simulink model "parameter_and_set_adaptation"  (R2020a)
settings: Solver=FixedStepAuto  StartTime=0.0  StopTime=ts  FixedStep=0.001  RelTol=1e-3
values from neighbouring files (symbols this model uses):
  eta = zeros(6,nt+1)    [run_Adaptive_Robust_MPCA.m]
  omega = zeros(size(x,1),size(theta,1),nt+1)    [run_Adaptive_Robust_MPCA.m]
  Q = zeros(size(Q0,1),size(Q0,2),nt+1)    [run_Adaptive_Robust_MPCA.m]
  thetaHat = zeros(3,nt+1)    [run_Adaptive_Robust_MPCA.m]
  V_e_eta = zeros(nt+1,1)    [run_Adaptive_Robust_MPCA.m]
  x = zeros(6,nt+1)    [run_Adaptive_Robust_MPCA.m]
  xHat = zeros(6,nt+1)    [run_Adaptive_Robust_MPCA.m]
undefined symbols (not defined in the file or in its folder): gamma, i, Ixx, Iyy, Izz, K, theta, z_theta0
settings Model: Creator=12894  LastModifiedBy=Maxwell
settings DebuggingCC: ArithmeticOperatorsInVariantConditions=warning
settings SFSimCC: CustomCodeUndefinedFunction=UseInterfaceOnly
settings CodeAppCC: StateflowObjectComments=on

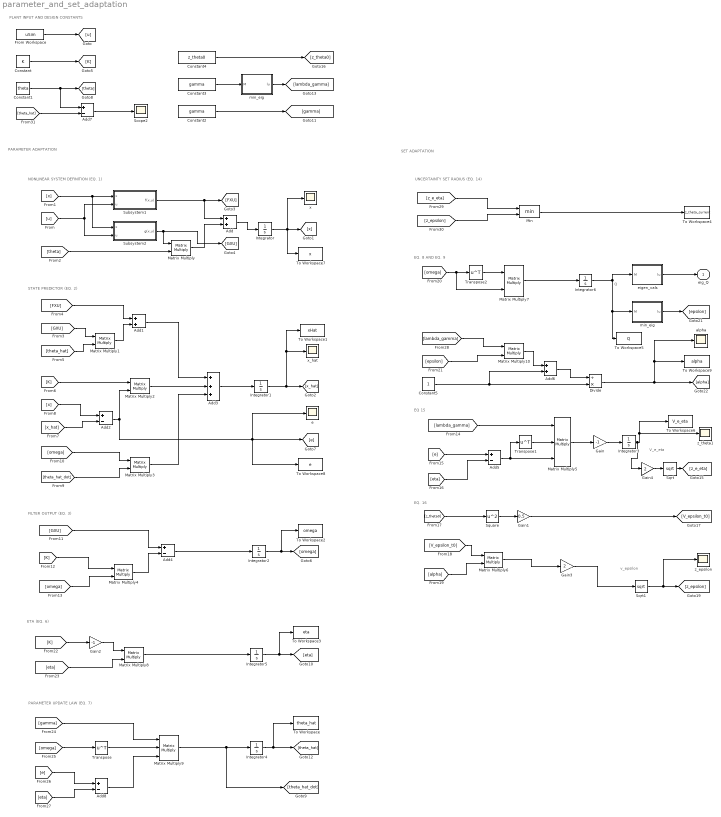
== system parameter_and_set_adaptation ==
  note: Q
  note: v_epsilon
  note: V_e_eta
  note: SET ADAPTATION
  note: UNCERTAINTY SET RADIUS (EQ. 14)
  note: EQ. 8 AND EQ. 9
  note: EQ. 16
  note: EQ 15
  note: PARAMETER ADAPTATION
  note: ETA (EQ. 6)
  note: PARAMETER UPDATE LAW (EQ. 7)
  note: FILTER OUTPUT (EQ. 3)
  note: STATE PREDICTOR (EQ. 2)
  note: NONLINEAR SYSTEM DEFINITION (EQ. 1)
  note: PLANT INPUT AND DESIGN CONSTANTS
  Add : Sum
  Add1 : Sum
  Add{2,4..5,7..8} (5 alike) : Sum  Inputs=+-
  Add3 : Sum  Inputs=+++
  Add6 : Sum
  Constant : Constant  Value=K
  Constant1 : Constant  Value=theta
  Constant2 : Constant  Value=gamma
  Constant3 : Constant  Value=gamma
  Constant4 : Constant  Value=z_theta0
  Constant5 : Constant
  Divide : Product  Inputs=/*
  From Workspace : FromWorkspace  VariableName=uSim
  Gain : Gain  Gain=-1
  Gain1 : Gain  Gain=0.5
  Gain2 : Gain  Gain=-1
  Gain3 : Gain  Gain=2
  Gain4 : Gain  Gain=2
  Integrator : Integrator  InitialCondition=x(:,i)
  Integrator1 : Integrator  InitialCondition=xHat(:,i)
  Integrator2 : Integrator  InitialCondition=omega(:,:,i)
  Integrator3 : Integrator  InitialCondition=V_e_eta(i)
  Integrator4 : Integrator  InitialCondition=thetaHat(:,i)
  Integrator5 : Integrator  InitialCondition=eta(:,i)
  Integrator6 : Integrator  InitialCondition=Q(:,:,i)
  Matrix Multiply{,1..4,6..8,10} (9 alike) : Product  Multiplication=Matrix(*)
  Matrix Multiply5 : Product  Inputs=3  Multiplication=Matrix(*)
  Matrix Multiply9 : Product  Inputs=3  Multiplication=Matrix(*)
  Min : MinMax  Inputs=2
  Scope2 : Scope
  Sqrt : Sqrt  SaturateOnIntegerOverflow=on
  Sqrt1 : Sqrt  SaturateOnIntegerOverflow=on
  Square : Math  Operator=square  SignedPower=on  SaturateOnIntegerOverflow=on
  Subsystem1 : Subsystem
  Subsystem2 : Subsystem
  To Workspace : ToWorkspace  VariableName=theta_hat  SaveFormat=Timeseries  SampleTime=-1
  To Workspace1 : ToWorkspace  VariableName=xHat  SaveFormat=Timeseries  SampleTime=-1
  To Workspace2 : ToWorkspace  VariableName=omega  SaveFormat=Timeseries  SampleTime=-1
  To Workspace3 : ToWorkspace  VariableName=eta  SaveFormat=Timeseries  SampleTime=-1
  To Workspace4 : ToWorkspace  VariableName=z_theta_current  SaveFormat=Timeseries  SampleTime=-1
  To Workspace5 : ToWorkspace  VariableName=Q  SaveFormat=Timeseries  SampleTime=-1
  To Workspace6 : ToWorkspace  VariableName=V_e_eta  SaveFormat=Timeseries  SampleTime=-1
  To Workspace7 : ToWorkspace  VariableName=x  SaveFormat=Timeseries  SampleTime=-1
  To Workspace8 : ToWorkspace  VariableName=e  SaveFormat=Timeseries  SampleTime=-1
  To Workspace9 : ToWorkspace  VariableName=alpha  SaveFormat=Timeseries  SampleTime=-1
  Transpose : Math  Operator=transpose  SignedPower=on  SaturateOnIntegerOverflow=on
  Transpose1 : Math  Operator=transpose  SignedPower=on  SaturateOnIntegerOverflow=on
  Transpose2 : Math  Operator=transpose  SignedPower=on  SaturateOnIntegerOverflow=on
  alpha : Scope
  e : Scope
  eigen_vals : MATLAB Function  TreatAsAtomicUnit=on
  min_eig : MATLAB Function  TreatAsAtomicUnit=on
  "min_eig " : MATLAB Function  TreatAsAtomicUnit=on
  x : Scope
  x_hat : Scope
  z_epsilon : Scope
  z_theta1 : Scope
  eig_Q : Outport  VectorParamsAs1DForOutWhenUnconnected=off
  wires:
  From Workspace/1 -> [u]
  [u] -> Subsystem1/2(u), Subsystem2/2(u)
  [x] -> Subsystem2/1(x), Subsystem1/1(x)
  Subsystem2/1(g(x,u)) -> [GXU], Matrix Multiply/1
  [theta] -> Matrix Multiply/2
  Subsystem1/1(f(x,u)) -> [FXU], Add/1
  Matrix Multiply/1 -> Add/2
  Integrator/1 -> To Workspace7/1, x/1, [x]
  Add/1 -> Integrator/1
  Matrix Multiply1/1 -> Add1/2
  [theta_hat] -> Matrix Multiply1/2
  Integrator1/1 -> To Workspace1/1, x_hat/1, [x_hat]
  [GXU] -> Matrix Multiply1/1
  [FXU] -> Add1/1
  [K] -> Matrix Multiply2/1
  Constant/1 -> [K]
  [x] -> Add2/1
  [x_hat] -> Add2/2
  Add2/1 -> To Workspace8/1, e/1, [e], Matrix Multiply2/2
  [omega] -> Matrix Multiply3/1
  [theta_hat_dot] -> Matrix Multiply3/2
  Add1/1 -> Add3/1
  Matrix Multiply2/1 -> Add3/2
  Matrix Multiply3/1 -> Add3/3
  Add3/1 -> Integrator1/1
  Integrator2/1 -> To Workspace2/1, [omega]
  [K] -> Matrix Multiply4/1
  [omega] -> Matrix Multiply4/2
  [GXU] -> Add4/1
  Matrix Multiply4/1 -> Add4/2
  Add4/1 -> Integrator2/1
  Constant1/1 -> Add7/1, [theta]
  Matrix Multiply8/1 -> Integrator5/1
  [eta] -> Matrix Multiply8/2
  Constant2/1 -> [gamma]
  [omega] -> Transpose/1
  [e] -> Add8/1
  [eta] -> Add8/2
  [gamma] -> Matrix Multiply9/1
  Transpose/1 -> Matrix Multiply9/2
  Add8/1 -> Matrix Multiply9/3
  Matrix Multiply9/1 -> [theta_hat_dot], Integrator4/1
  Integrator4/1 -> To Workspace/1, [theta_hat]
  Integrator5/1 -> To Workspace3/1, [eta]
  [eta] -> Add5/2
  [e] -> Add5/1
  [lambda_gamma] -> Matrix Multiply5/1
  Transpose1/1 -> Matrix Multiply5/2
  Add5/1 -> Matrix Multiply5/3, Transpose1/1
  Constant3/1 -> "min_eig "/1(M)
  Matrix Multiply5/1 -> Gain/1
  Gain/1 -> Integrator3/1
  Sqrt/1 -> [z_e_eta]
  Constant4/1 -> [z_theta0]
  [z_theta0] -> Square/1
  Square/1 -> Gain1/1
  Gain1/1 -> [V_epsilon_t0]
  [V_epsilon_t0] -> Matrix Multiply6/1
  [alpha] -> Matrix Multiply6/2
  Sqrt1/1 -> z_epsilon/1, [z_epsilon]
  Transpose2/1 -> Matrix Multiply7/1
  [omega] -> Matrix Multiply7/2, Transpose2/1
  Matrix Multiply7/1 -> Integrator6/1
  Integrator6/1 -> eigen_vals/1(M), To Workspace5/1, min_eig/1(M)
  [lambda_gamma] -> Matrix Multiply10/1
  [epsilon] -> Matrix Multiply10/2
  Matrix Multiply10/1 -> Add6/1
  Constant5/1 -> Divide/2, Add6/2
  Add6/1 -> Divide/1
  Divide/1 -> To Workspace9/1, alpha/1, [alpha]
  [z_e_eta] -> Min/1
  [z_epsilon] -> Min/2
  Min/1 -> To Workspace4/1
  min_eig/1(lu) -> [epsilon]
  "min_eig "/1(lu) -> [lambda_gamma]
  [theta_hat] -> Add7/2
  Add7/1 -> Scope2/1
  eigen_vals/1(lu) -> eig_Q/1
  [K] -> Gain2/1
  Gain2/1 -> Matrix Multiply8/1
  Matrix Multiply6/1 -> Gain3/1
  Gain3/1 -> Sqrt1/1
  Gain4/1 -> Sqrt/1
  Integrator3/1 -> Gain4/1, To Workspace6/1, z_theta1/1

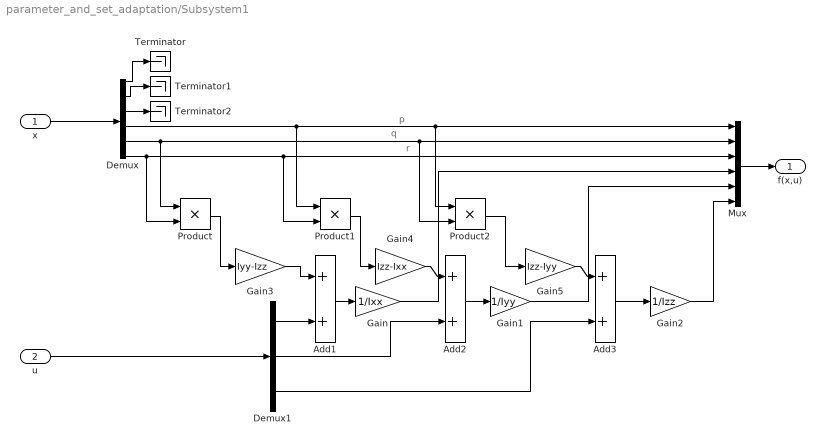
== system parameter_and_set_adaptation/Subsystem1 ==
  note: p
  note: q
  note: r
  x : Inport
  u : Inport  Port=2
  Add1 : Sum
  Add2 : Sum
  Add3 : Sum
  Demux : Demux  Outputs=6
  Demux1 : Demux  Outputs=3
  Gain : Gain  Gain=1/Ixx
  Gain1 : Gain  Gain=1/Iyy
  Gain2 : Gain  Gain=1/Izz
  Gain3 : Gain  Gain=Iyy-Izz
  Gain4 : Gain  Gain=Izz-Ixx
  Gain5 : Gain  Gain=Izz-Iyy
  Mux : Mux  Inputs=6
  Product : Product
  Product1 : Product
  Product2 : Product
  Terminator : Terminator
  Terminator1 : Terminator
  Terminator2 : Terminator
  f(x,u) : Outport  VectorParamsAs1DForOutWhenUnconnected=off
  wires:
  x/1 -> Demux/1
  Mux/1 -> f(x,u)/1
  Demux/5 -> Product/1, Product2/2, Mux/2
  Demux/6 -> Product/2, Product1/2, Mux/3
  Demux/1 -> Terminator/1
  Demux/2 -> Terminator1/1
  Demux/3 -> Terminator2/1
  u/1 -> Demux1/1
  Demux/4 -> Product2/1, Mux/1, Product1/1
  Product/1 -> Gain3/1
  Product1/1 -> Gain4/1
  Product2/1 -> Gain5/1
  Gain3/1 -> Add1/1
  Gain4/1 -> Add2/1
  Gain5/1 -> Add3/1
  Demux1/1 -> Add1/2
  Demux1/2 -> Add2/2
  Demux1/3 -> Add3/2
  Add1/1 -> Gain/1
  Add2/1 -> Gain1/1
  Add3/1 -> Gain2/1
  Gain/1 -> Mux/4
  Gain1/1 -> Mux/5
  Gain2/1 -> Mux/6

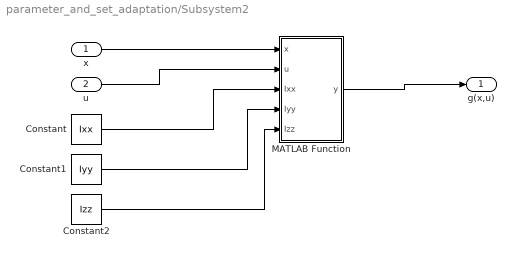
== system parameter_and_set_adaptation/Subsystem2 ==
  x : Inport
  u : Inport  Port=2
  Constant : Constant  Value=Ixx
  Constant1 : Constant  Value=Iyy
  Constant2 : Constant  Value=Izz
  MATLAB Function : MATLAB Function  TreatAsAtomicUnit=on
  g(x,u) : Outport  VectorParamsAs1DForOutWhenUnconnected=off
  wires:
  x/1 -> MATLAB Function/1(x)
  u/1 -> MATLAB Function/2(u)
  MATLAB Function/1(y) -> g(x,u)/1
  Constant/1 -> MATLAB Function/3(Ixx)
  Constant1/1 -> MATLAB Function/4(Iyy)
  Constant2/1 -> MATLAB Function/5(Izz)

== matlab function parameter_and_set_adaptation/min_eig  ==
  data: M input; lu output
function lu = min_eig(M)
lu = min(real(eig(M)));

== matlab function parameter_and_set_adaptation/min_eig ==
  data: M input; lu output
function lu = min_eig(M)
lu = min(real(eig(M)));

== matlab function parameter_and_set_adaptation/eigen_vals ==
  data: M input; lu output
function lu = eigen_vals(M)
lu = eig(M);

== matlab function parameter_and_set_adaptation/Subsystem2/MATLAB Function ==
  data: x input; u input; y output; Ixx input; Iyy input; Izz input
function y = gxu(x, u, Ixx, Iyy, Izz)
    y = zeros(6,3);
    
    y(4,1) = 1/Ixx;
    y(5,2) = 1/Iyy;
    y(6,3) = 1/Izz;
end
